simulink model "singlemcu"  (R2025a)
settings: Solver=VariableStepAuto  StartTime=0.0  StopTime=5  RelTol=1e-3
libraries: statsLibrary x1, dspvision x1, audiofeatures x1
settings Model: Creator=DELL  LastModifiedBy=DELL

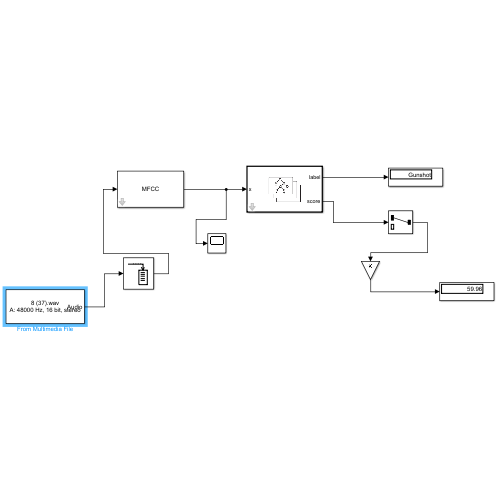
[thumbnail: Simulink's stored preview of the top-level diagram]
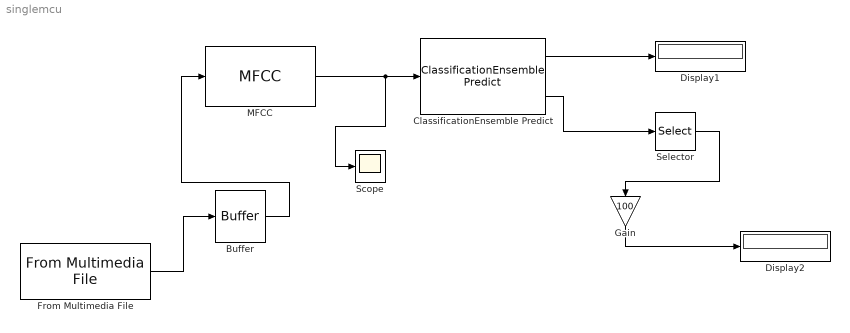
== system singlemcu ==
  Buffer : Buffer  N=88200  V=44100  OutputFrames=off
  ClassificationEnsemble Predict : statsLibrary/Classification/ClassificationEnsemble Predict  TrainedLearner=trainedModel  ShowOutputScore=on  LabelOutMin=[]  LabelOutMax=[]  ScoreOutMin=[]  ScoreOutMax=[]  RawScoreOutMin=[]  RawScoreOutMax=[]  WeakLearnerOutMin=[]  WeakLearnerOutMax=[]  StoredEnumName=trainedModel_enumLabels
  Display1 : Display
  Display2 : Display
  From Multimedia File : dspvision/From Multimedia File  inputFilename=D:\linearalgebra\Data\Gunshot\8 (37).wav  readRange=[1 Inf]  loop=on  numPlays=inf  outputStreams=Audio only  videoDataType=single  audioDataType=double  inheritSampleTime=on  userDefinedSampleTime=1/30  noAudioOutput=off  isIntensityVideo=off  fourcc=RGB  colorVideoFormat=Separate color signals  outputEOF=off  dataOrg=Column-major  audioFrameSize=1024  computeAudioFrameSize=off  outSamplingMode=Sample based
      settings: LibrarySourceBlock=audiosources/From Multimedia File
  Gain : Gain  Gain=100
  MFCC : audiofeatures/MFCC  WindowParameter=hamming(1024,'periodic')  OverlapLength=512  NumCoeffs=13  Rectification=Logarithm  AppendDelta=off  AppendDeltaDelta=off  DeltaWindowLength=9  NumFeatureVectors=1  NumFeatureVectorOverlap=0  InheritSampleRate=on  SampleRate=44.1e3  NumBands=32  AutoFrequencyRange=on  FrequencyRange=[0, 22050]  FilterBankDesignDomain=linear  FilterBankNormalization=bandwidth  MelStyle=oshaughnessy  WindowNormalization=on  SpectrumType=power  AutoFFTLength=on  FFTLength=1024
  Scope : Scope
      settings: ActiveDisplayYMinimum=-2053.6294815911597  ActiveDisplayYMaximum=357.80029529195144
  Selector : Selector  InputPortWidth=2  IndexOptions=Index vector (dialog)  Indices=1  OutputSizes=1
  wires:
  Gain/1 -> Display2/1
  Selector/1 -> Gain/1
  ClassificationEnsemble Predict/2 -> Selector/1
  ClassificationEnsemble Predict/1 -> Display1/1
  Buffer/1 -> MFCC/1
  MFCC/1 -> ClassificationEnsemble Predict/1, Scope/1
  From Multimedia File/1 -> Buffer/1
